simulink model "project"  (R2017a)
settings: Solver=VariableStepAuto  StartTime=0.0  StopTime=100  RelTol=1e-3
values from neighbouring files (symbols this model uses):
  A = [0    1    0    0;0    -2*(cf+cr)/(m*vx)    2*(cf+cr)/m     -(2*a*cf-2*b*cr)/(m*vx);0     0     0    1;0     -(2*a*cf-2*b*cr)/(iz*vx)    (2*a*cf-2*b*cr)/iz    -(2*a^2*cf+2*b^2*cr)/(iz*vx)]    [MIMO.m]    (also in SISO.m)
  B = [0 0;2*cf/m -(2*a*cf-2*b*cr)/(m*vx)-vx;0 0;2*a*cf/iz -(2*a^2*cf+2*b^2*cr)/(iz*vx)]    [MIMO.m]    (also in SISO.m = [0 ;2*cf/m ;0 ;2*a*cf/iz ])
  C = [1 0 0 0]    [MIMO.m]    (also in SISO.m)
  gain = 1/G_cl    [SISO.m]
  k = [k11 k12 k13 k14;k21 k22 k23 k24]    [MIMO.m]    (also in SISO.m = (alphak-ak)*inv(psi)*inv(phi_c))
  k_int2 = k_int(5)    [SISO.m]
  L = [8.6078; 15.729; 3.191; -25.568]    [SISO.m]
undefined symbols (not defined in the file or in its folder): k_int1
libraries: simulink x1
settings Model: Creator=Administrator  LastModifiedBy=Administrator

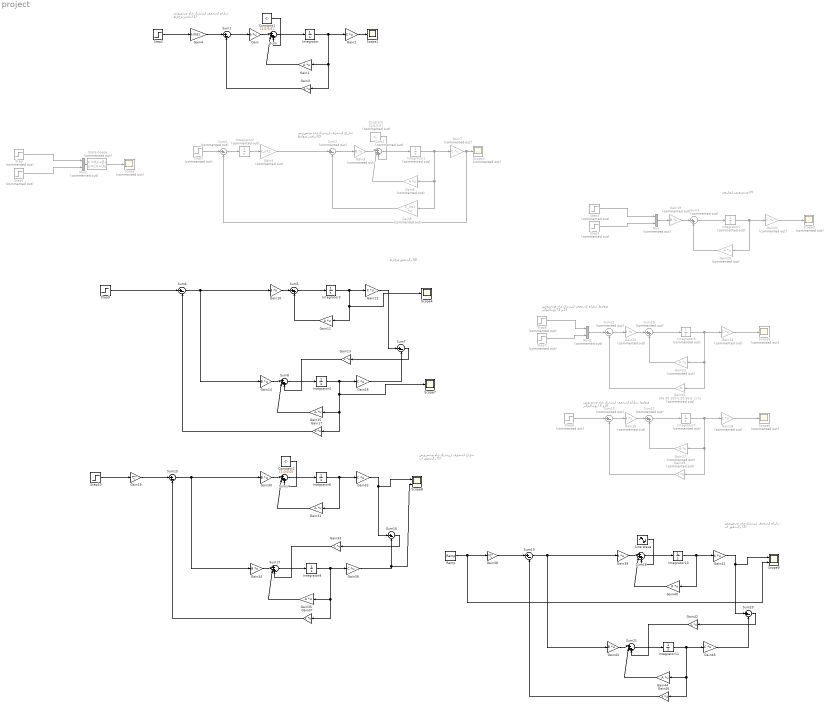
== system project ==
  note: سیستم های کنترل فیدبک حالت با رویتگر (2)
  note: سیستم های کنترل فیدبک حالت با رویتگر (1)
  note: تحلیل سیستم(7)
  note: طراحی رویتگر (4)
  note: سیستم های کنترل فیدبک حالت: طراحی ردیاب(2)
  note: سیستم های کنترل فیدبک حالت: طراحی ردیاب(1)
  note: سیستم های کنترل فیدبک حالت: طراحی رگولاتور (3 و 4)
  note: سیستم های کنترل فیدبک حالت: طراحی رگولاتور (1 و 2)
  Constant : Constant  Commented=on  Value=[1;0;0;0]
  Constant1 : Constant  Value=[1;0;0;0]
  Constant2 : Constant  Value=[1;0;0;0]
  Gain{,10,14,30,34,39,43} (7 alike) : Gain  Gain=B  Multiplication=Matrix(K*u)
  Gain{1,11,15,31,35,40,44} (7 alike) : Gain  Gain=A  Multiplication=Matrix(K*u)
  Gain{2,12,16,32,36,41,45} (7 alike) : Gain  Gain=C  Multiplication=Matrix(K*u)
  Gain13 : Gain  Gain=L  Multiplication=Matrix(K*u)
  Gain{3,17,37,46} (4 alike) : Gain  Gain=k  Multiplication=Matrix(K*u)
  Gain18 : Gain  Gain=gain  Multiplication=Matrix(K*u)
  Gain{5,19,22,26} (4 alike) : Gain  Commented=on  Gain=B  Multiplication=Matrix(K*u)
  Gain{6,20,23,27} (4 alike) : Gain  Commented=on  Gain=A  Multiplication=Matrix(K*u)
  Gain{7,21,24,28} (4 alike) : Gain  Commented=on  Gain=C  Multiplication=Matrix(K*u)
  Gain25 : Gain  Commented=on  Gain=[45 30 100 6;20 50 6 1]  Multiplication=Matrix(K*u)
  Gain29 : Gain  Commented=on  Gain=k  Multiplication=Matrix(K*u)
  Gain33 : Gain  Gain=L  Multiplication=Matrix(K*u)
  Gain38 : Gain  Gain=gain  Multiplication=Matrix(K*u)
  Gain4 : Gain  Gain=0.0031
  Gain42 : Gain  Gain=L  Multiplication=Matrix(K*u)
  Gain8 : Gain  Commented=on  Gain=k_int1  Multiplication=Matrix(K*u)
  Gain9 : Gain  Commented=on  Gain=k_int2
  Integrator{,4,9,11} (4 alike) : Integrator
  Integrator{1..2,5..6} (4 alike) : Integrator  Commented=on
  Integrator10 : Integrator  InitialCondition=[1;0;0;0]
  Integrator3 : Integrator  InitialCondition=[1;0;0;0]
  Integrator7 : Integrator  Commented=on  InitialCondition=[1; 1; 0 ;0]
  Integrator8 : Integrator  InitialCondition=[1;0;0;0]
  Mux : Mux  Commented=on  Inputs=2
  Mux1 : Mux  Commented=on  Inputs=2
  Mux2 : Mux  Commented=on  Inputs=2
  Ramp : simulink/Sources/Ramp  slope=1  start=0  X0=0
  Scope{,2..3,5..6} (5 alike) : Scope  Commented=on
  Scope1 : Scope
  Scope4 : Scope
  Scope7 : Scope
  Scope8 : Scope  NumInputPorts=2
  Scope9 : Scope  NumInputPorts=2
  Sine Wave : Sin  Frequency=1/pi  SampleTime=0
  State-Space : StateSpace  Commented=on  A=A  B=B  C=C  D=[0 0]  X0=0
  Step{,1,3..8} (8 alike) : Step  Commented=on  SampleTime=0
  Step10 : Step  SampleTime=0
  Step2 : Step  SampleTime=0
  Step9 : Step  After=0  SampleTime=0
  Sum{,8,14,17..18,21} (6 alike) : Sum  Inputs=|+++
  Sum{1,6..7,15..16,19..20} (7 alike) : Sum  Inputs=|+-
  Sum10 : Sum  Commented=on  Inputs=|++
  Sum{3..4,11,13} (4 alike) : Sum  Commented=on  Inputs=|+-
  Sum12 : Sum  Commented=on  Inputs=|++
  Sum2 : Sum  Commented=on  Inputs=|+++
  Sum5 : Sum  Inputs=|++
  Sum9 : Sum  Commented=on  Inputs=|++
  wires:
  State-Space/1 -> Scope/1
  Mux1/1 -> State-Space/1
  Step/1 -> Mux1/1
  Step1/1 -> Mux1/2
  Gain/1 -> Sum/1
  Gain1/1 -> Sum/2
  Step2/1 -> Gain4/1
  Gain4/1 -> Sum1/1
  Sum1/1 -> Gain/1
  Gain3/1 -> Sum1/2
  Sum/1 -> Integrator/1
  Integrator/1 -> Gain3/1, Gain1/1, Gain2/1
  Gain2/1 -> Scope1/1
  Gain9/1 -> Sum3/1
  Sum3/1 -> Gain5/1
  Gain8/1 -> Sum3/2
  Gain7/1 -> Sum4/2, Scope2/1
  Integrator1/1 -> Gain8/1, Gain6/1, Gain7/1
  Gain6/1 -> Sum2/2
  Gain5/1 -> Sum2/1
  Sum2/1 -> Integrator1/1
  Sum4/1 -> Integrator2/1
  Integrator2/1 -> Gain9/1
  Step3/1 -> Sum4/1
  Gain10/1 -> Sum5/1
  Sum6/1 -> Gain14/1, Gain10/1
  Sum5/1 -> Integrator3/1
  Integrator3/1 -> Scope4/1, Gain11/1, Gain12/1
  Gain11/1 -> Sum5/2
  Gain12/1 -> Sum7/1
  Sum7/1 -> Gain13/1
  Gain14/1 -> Sum8/1
  Gain15/1 -> Sum8/2
  Sum8/1 -> Integrator4/1
  Integrator4/1 -> Scope7/1, Gain17/1, Gain15/1, Gain16/1
  Gain16/1 -> Sum7/2
  Gain13/1 -> Sum8/3
  Gain17/1 -> Sum6/2
  Step9/1 -> Sum6/1
  Integrator5/1 -> Gain20/1, Gain21/1
  Gain20/1 -> Sum9/2
  Sum9/1 -> Integrator5/1
  Gain19/1 -> Sum9/1
  Gain21/1 -> Scope3/1
  Step4/1 -> Mux/1
  Step5/1 -> Mux/2
  Mux/1 -> Gain19/1
  Gain22/1 -> Sum10/1
  Sum10/1 -> Integrator6/1
  Gain23/1 -> Sum10/2
  Integrator6/1 -> Gain25/1, Gain23/1, Gain24/1
  Step6/1 -> Mux2/1
  Step7/1 -> Mux2/2
  Gain24/1 -> Scope5/1
  Gain25/1 -> Sum11/2
  Sum11/1 -> Gain22/1
  Mux2/1 -> Sum11/1
  Sum13/1 -> Gain26/1
  Gain27/1 -> Sum12/2
  Integrator7/1 -> Gain29/1, Gain27/1, Gain28/1
  Gain28/1 -> Scope6/1
  Sum12/1 -> Integrator7/1
  Gain26/1 -> Sum12/1
  Gain29/1 -> Sum13/2
  Step8/1 -> Sum13/1
  Constant/1 -> Sum2/3
  Constant1/1 -> Sum/3
  Gain35/1 -> Sum17/2
  Sum16/1 -> Gain33/1
  Sum14/1 -> Integrator8/1
  Gain30/1 -> Sum14/1
  Gain32/1 -> Scope8/1, Sum16/1
  Integrator8/1 -> Gain31/1, Gain32/1
  Gain36/1 -> Scope8/2, Sum16/2
  Gain31/1 -> Sum14/2
  Gain37/1 -> Sum15/2
  Sum17/1 -> Integrator9/1
  Sum15/1 -> Gain34/1, Gain30/1
  Gain34/1 -> Sum17/1
  Gain33/1 -> Sum17/3
  Integrator9/1 -> Gain37/1, Gain35/1, Gain36/1
  Constant2/1 -> Sum14/3
  Step10/1 -> Gain18/1
  Gain18/1 -> Sum15/1
  Integrator11/1 -> Gain46/1, Gain44/1, Gain45/1
  Sum21/1 -> Integrator11/1
  Sum19/1 -> Gain43/1, Gain39/1
  Gain43/1 -> Sum21/1
  Gain46/1 -> Sum19/2
  Gain45/1 -> Sum20/2
  Integrator10/1 -> Gain40/1, Gain41/1
  Gain41/1 -> Scope9/1, Sum20/1
  Gain40/1 -> Sum18/2
  Gain39/1 -> Sum18/1
  Sum20/1 -> Gain42/1
  Gain44/1 -> Sum21/2
  Ramp/1 -> Scope9/2, Gain38/1
  Sum18/1 -> Integrator10/1
  Gain42/1 -> Sum21/3
  Gain38/1 -> Sum19/1
  Sine Wave/1 -> Sum18/3
